simulink model "Differential"  (R2023b)
settings: Solver=VariableStepAuto  StartTime=0.0  StopTime=30.0  RelTol=1e-3
settings Model: Creator=Hirbod  LastModifiedBy=Hirbod

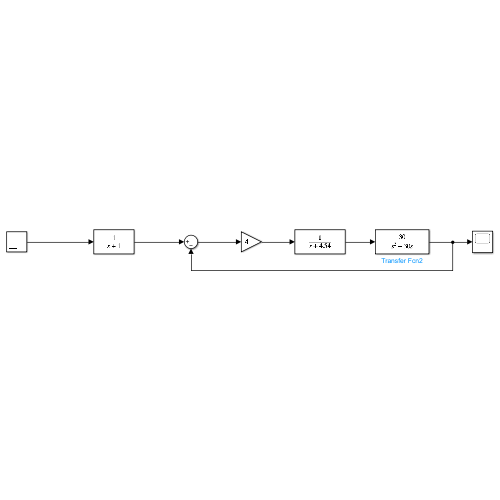
[thumbnail: Simulink's stored preview of the top-level diagram]
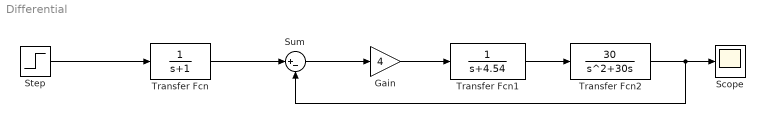
== system Differential ==
  Gain : Gain  Gain=4
  Scope : Scope
  Step : Step  After=30  SampleTime=0
  Sum : Sum  Inputs=|+-
  Transfer Fcn : TransferFcn  Denominator=[1 1]
  Transfer Fcn1 : TransferFcn  Denominator=[1 4.54]
  Transfer Fcn2 : TransferFcn  Numerator=[30]  Denominator=[1 30 0]
  wires:
  Step/1 -> Transfer Fcn/1
  Sum/1 -> Gain/1
  Transfer Fcn/1 -> Sum/1
  Gain/1 -> Transfer Fcn1/1
  Transfer Fcn1/1 -> Transfer Fcn2/1
  Transfer Fcn2/1 -> Sum/2, Scope/1
